simulink model "continuousProcess"  (R2020b)
settings: Solver=VariableStepAuto  StartTime=0.0  StopTime=250.0  RelTol=1e-3
libraries: fuzblock x1
settings Model: Creator=sergio  LastModifiedBy=sergio

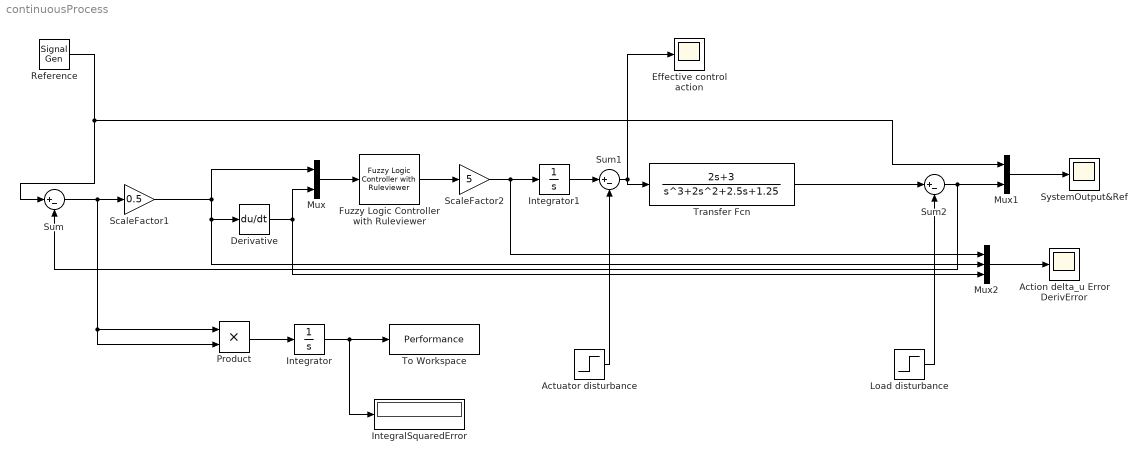
== system continuousProcess ==
  Action delta_u Error DerivError : Scope
  Actuator disturbance : Step  Time=75  After=0  SampleTime=0
  "Derivative " : Derivative
  Effective control action : Scope
  Fuzzy Logic Controller with Ruleviewer : fuzblock/Fuzzy Logic  Controller  with Ruleviewer  fismatrix=fuzzySystem  Ts=2
  IntegralSquaredError : Display
  Integrator : Integrator
  Integrator1 : Integrator
  Load disturbance : Step  Time=150  After=0  SampleTime=0
  Mux : Mux  Inputs=2
  Mux1 : Mux  Inputs=2
  Mux2 : Mux  Inputs=3
  Product : Product
  Reference : SignalGenerator  WaveForm=square  Frequency=0.05  Units=rad/sec
  ScaleFactor1 : Gain  Gain=0.5
  ScaleFactor2 : Gain  Gain=5
  Sum : Sum  Inputs=|+-
  Sum1 : Sum  Inputs=|+-
  Sum2 : Sum  Inputs=|+-
  SystemOutput&Ref : Scope
  To Workspace : ToWorkspace  VariableName=Performance  SaveFormat=Timeseries  SampleTime=-1
  Transfer Fcn : TransferFcn  Numerator=[2 3]  Denominator=[1 2 2.5 1.25]
  wires:
  ScaleFactor1/1 -> Mux/1, Mux2/2, "Derivative "/1
  ScaleFactor2/1 -> Mux2/1, Integrator1/1
  Mux2/1 -> Action delta_u Error DerivError/1
  Mux1/1 -> SystemOutput&Ref/1
  Integrator/1 -> IntegralSquaredError/1, To Workspace/1
  "Derivative "/1 -> Mux/2, Mux2/3
  Reference/1 -> Sum/1, Mux1/1
  Integrator1/1 -> Sum1/1
  Fuzzy Logic Controller with Ruleviewer/1 -> ScaleFactor2/1
  Product/1 -> Integrator/1
  Transfer Fcn/1 -> Sum2/1
  Sum/1 -> Product/2, Product/1, ScaleFactor1/1
  Mux/1 -> Fuzzy Logic Controller with Ruleviewer/1
  Load disturbance/1 -> Sum2/2
  Sum2/1 -> Mux1/2, Sum/2
  Actuator disturbance/1 -> Sum1/2
  Sum1/1 -> Effective control action/1, Transfer Fcn/1
